simulink model "henon2d"  (Simulink 3.00)
settings: Solver=ode45  SolverMode=SingleTasking  StartTime=0.0  StopTime=100  RelTol=1e-3  AbsTol=1e-6
undefined symbols (not defined in the file or in its folder): sfunxyzd
settings Model: ExternalInput=[]  SaveTime=off  SaveOutput=off  InitialState=[]  IntegerOverflowMsg=none  RTWOptions="-aEnforceIntegerDowncast=1 -aFoldNonRolledExpr=1 -aInlineInvariantSignals=1 -aInlineParameters=0 -aLocalBlockOutputs=1 -aRollThreshold=5 -aZeroInternalMemoryAtStartup=1 -aZeroExternalMemoryAtStartup=1 -aInitFltsAndDblsToZero=1 -aGenerateReport=0 -aGenCodeOnly=0 -aRTWVerbose=1 -aIncludeHyperlinkInReport=0 -aLaunchReport=0 -aForceParamTrailComments=0 -aGenerateComments=1 -aIgnoreCustomStorageClasses=1 -aIncHierarchyInIds=0 -aMaxRTWIdLen=31 -aShowEliminatedStatements=0 -aPrefixModelToSubsysFcnNames=1 -aIncDataTypeInIds=0 -aInsertBlockDesc=0 -aSimulinkBlockComments=1 -aInlinedPrmAccess=\"Literals\"  -aSuppressErrorStatus=0 -aModelReferenceCompliant=1 -aSupportNonInlinedSFcns=1 -aSupportContinuousTime=1 -aSupportComplex=1 -aSupportNonFinite=1 -aSupportAbsoluteTime=1 -aTargetFcnLib=\"ansi_tfl_tmw.mat\" -aMultiInstanceERTCode=0 -aLogVarNameModifier=\"rt_\" -aIsPILTarget=0 -aCombineOutputUpdateFcns=0 -aGenerateASAP2=0 -aGenerateSampleERTMain=0 -aGenerateFullHeader=1 -aUtilityFuncGeneration=\"Auto\" -aIncludeFileDelimiter=\"Auto\" -aIncludeMdlTerminateFcn=1 -aPurelyIntegerCode=0 -aERTCustomFileBanners=0 -aRTWCAPIStates=0 -aRTWCAPIParams=0 -aRTWCAPISignals=0 -aMatFileLogging=1 -aGenFloatMathFcnCalls=\"ANSI_C\" -aExtModeMexFile=\"ext_comm\" -aExtModeTransport=0 -aExtModeStaticAllocSize=1000000 -aExtModeTesting=0 -aExtModeStaticAlloc=0 -aExtMode=0  -aInitFltsAndDblsToZero=1 -aInitFltsAndDblsToZero=1"  Creator=The MathWorks Inc.  LastModifiedBy=campa

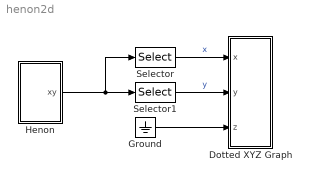
== system henon2d ==
  Dotted XYZ Graph : Subsystem  LoadFcn=sfunxyzd([],[],[],'LoadBlock')  StartFcn=sfunxyzd([],[],[],'Start')  StopFcn=sfunxyzd([],[],[],'Stop')  mask(XYZ multiscope (dots)){np=1, xlim=[-2 2], ylim=[-1 1]/2, zlim=[0 1], cp=[0 0 1], gd=on, st=0.02}
      mask prompts: np "Number of lines"; xlim "[xmin xmax]"; ylim "[ymin ymax]"; zlim "[zmin zmax]"; cp "Camera position (use [0 0 1] for 2D XY view)"; gd "Grid"; st "Sample time:"
      mask help:
      | Multidimensional XYZ dotted scope using MATLAB graph window.
      |    X,Y,Z coordinates are respectively the first,second, and third input.
      |    Enter the number of lines, the XYZ ranges, the camera position,
      |    and the sampling time, as mask parameters.
      settings: CopyFcn=sfunxyzd([],[],[],'CopyBlock')  DeleteFcn=sfunxyzd([],[],[],'DeleteBlock')  NameChangeFcn=sfunxyzd([],[],[],'NameChange')
      mask Help:
      | This block can be used to explore limit cycles.
      |    Look at the m-file sfunxyzd.m to see how it works.
      mask Display: plot([.05 .95 .95 .05 .05],[.45 .45 .95 .95 .45], 0.5+cos(0:0.1:2*pi)*0.3,0.7+sin(0:0.1:2*pi)*0.2)
  Ground : Ground
  Henon : Subsystem  mask(Henon System){a=1.4, b=0.3, xy0=[0 0], T=0.01}
      mask prompts: xy0 "Initial point p0 = [x0 y0]"; T "Sampling Time"
      mask help:
      | This autonomous system represents the henon equation:
      | xnew =  1 + y - a*x*x;  ynew =  b*x;
      | Parameters and initial state can be selected from the mask.
      mask Help:
      | This autonomous system represents the henon equation.
      | Parameters and initial state can be selected from the mask.
      | <p>
      | The system equations are:
      | xnew =  1 + y - a*x*x;
      | ynew =  b*x;
  Selector : Selector  Elements=1  InputPortWidth=2
  Selector1 : Selector  Elements=2  InputPortWidth=2
  wires:
  Henon/1(xy) -> Selector/1, Selector1/1
  Selector/1 -> Dotted XYZ Graph/1(x)  "x"
  Selector1/1 -> Dotted XYZ Graph/2(y)  "y"
  Ground/1 -> Dotted XYZ Graph/3(z)

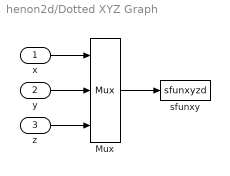
== system henon2d/Dotted XYZ Graph ==
  x : Inport  Port=1  PortWidth=-1  SampleTime=-1  DataType=auto
      settings: SignalType=auto
  y : Inport  Port=2  PortWidth=-1  SampleTime=-1  DataType=auto
      settings: SignalType=auto
  z : Inport  Port=3  PortWidth=-1  SampleTime=-1  DataType=auto
      settings: SignalType=auto
  Mux : Mux  Inputs=[np np np]
      settings: DisplayOption=none
  sfunxy : S-Function  FunctionName=sfunxyzd  Parameters=[xlim ylim zlim],st,np,cp,gd  PortCounts=[]  SFunctionModules=''
  wires:
  Mux/1 -> sfunxy/1
  x/1 -> Mux/1
  y/1 -> Mux/2
  z/1 -> Mux/3

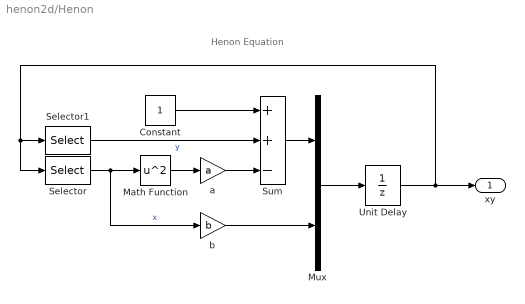
== system henon2d/Henon ==
  note: Henon Equation
  Constant : Constant  Value=1
  Math Function : Math  Operator=square  OutputSignalType=auto
  Mux : Mux  Inputs=[1 1]
  Selector : Selector  Elements=1  InputPortWidth=2
  Selector1 : Selector  Elements=2  InputPortWidth=2
  Sum : Sum  Inputs=++-  SaturateOnIntegerOverflow=on
  Unit Delay : UnitDelay  X0=xy0  SampleTime=T
  a : Gain  Gain=a  SaturateOnIntegerOverflow=on
  b : Gain  Gain=b  SaturateOnIntegerOverflow=on
  xy : Outport  Port=1
  wires:
  Math Function/1 -> a/1
  a/1 -> Sum/3
  Sum/1 -> Mux/1
  Constant/1 -> Sum/1
  Selector1/1 -> Sum/2  "y"
  Selector/1 -> Math Function/1, b/1  "x"
  b/1 -> Mux/2
  Mux/1 -> Unit Delay/1
  Unit Delay/1 -> xy/1, Selector1/1, Selector/1
